simulink model "malhaContinua"  (R2022b)
settings: Solver=VariableStepAuto  StartTime=0.0  StopTime=30  RelTol=1e-3
values from neighbouring files (symbols this model uses):
  disturbio = 0.24    [lab4.m]
  R = 1.18    [lab4.m]
undefined symbols (not defined in the file or in its folder): den, num
settings Model: Creator=mathe  LastModifiedBy=mathe

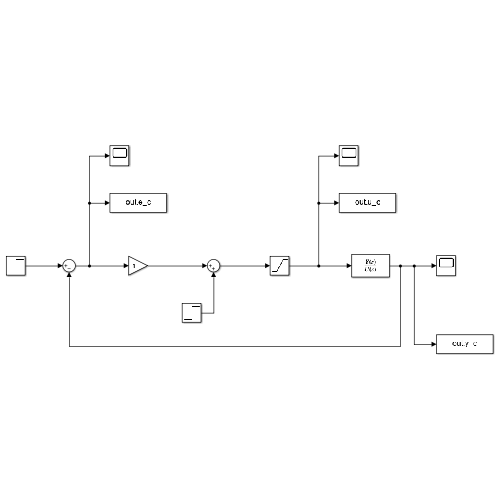
[thumbnail: Simulink's stored preview of the top-level diagram]
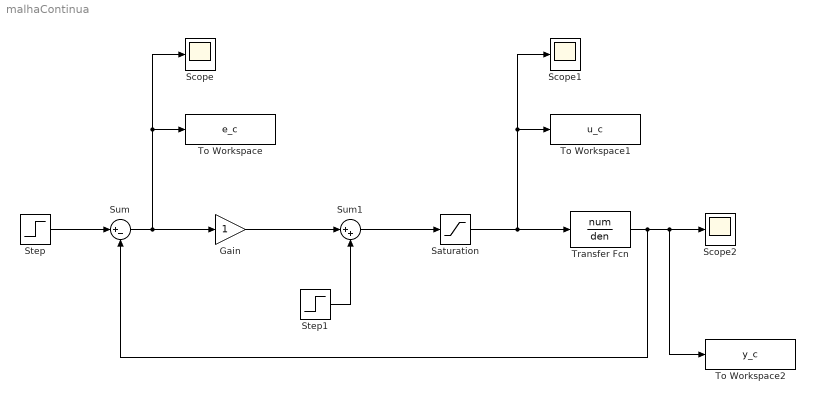
== system malhaContinua ==
  Gain : Gain
  Saturation : Saturate  UpperLimit=10  LowerLimit=-10
  Scope : Scope
  Scope1 : Scope
  Scope2 : Scope
  Step : Step  Time=0  After=R  SampleTime=0
  Step1 : Step  Time=15  After=disturbio  SampleTime=0
  Sum : Sum  Inputs=|+-
  Sum1 : Sum  Inputs=|++
  To Workspace : ToWorkspace  VariableName=e_c  SaveFormat=Timeseries  SampleTime=-1
  To Workspace1 : ToWorkspace  VariableName=u_c  SaveFormat=Timeseries  SampleTime=-1
  To Workspace2 : ToWorkspace  VariableName=y_c  SaveFormat=Timeseries  SampleTime=-1
  Transfer Fcn : TransferFcn  Numerator=num  Denominator=den
  wires:
  Gain/1 -> Sum1/1
  Sum/1 -> Scope/1, To Workspace/1, Gain/1
  Step/1 -> Sum/1
  Step1/1 -> Sum1/2
  Sum1/1 -> Saturation/1
  Saturation/1 -> Scope1/1, To Workspace1/1, Transfer Fcn/1
  Transfer Fcn/1 -> Sum/2, To Workspace2/1, Scope2/1
